simulink model "ex_longitudinal_force_balance"  (R2026a)
settings: Solver=VariableStepAuto
libraries: aerolibconvert2 x1
settings Model: Creator=doyeop  LastModifiedBy=doyeop

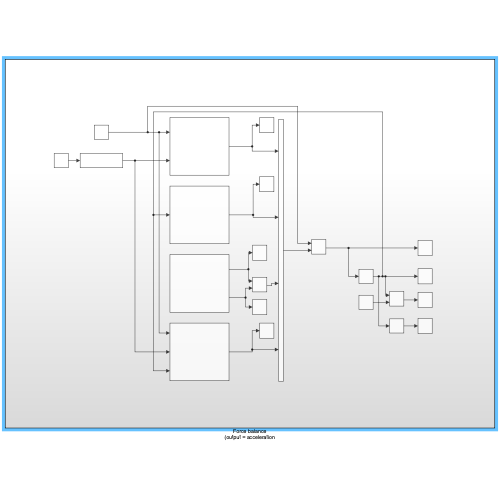
[thumbnail: Simulink's stored preview of the top-level diagram]
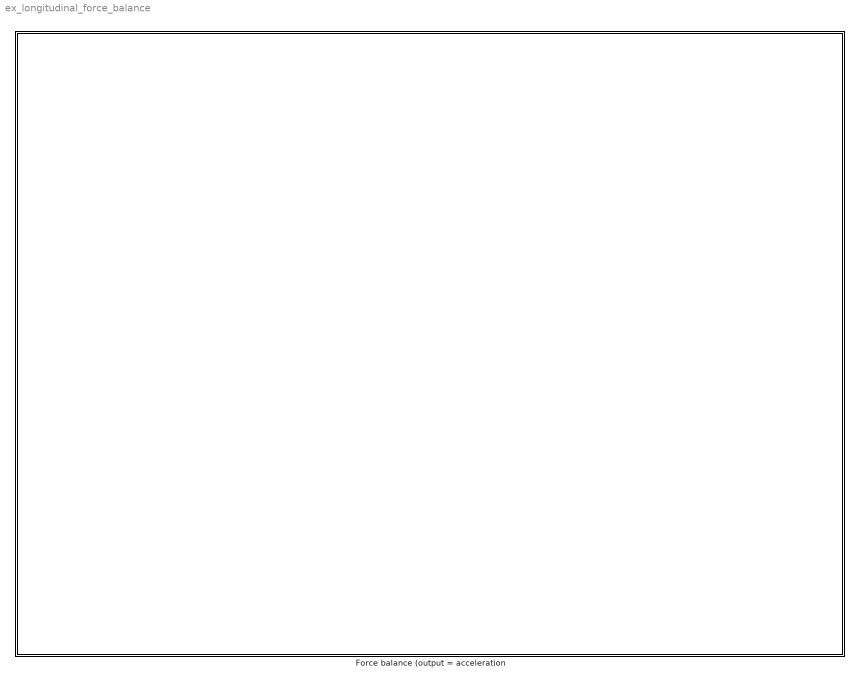
== system ex_longitudinal_force_balance ==
  Force balance (output = acceleration : Subsystem

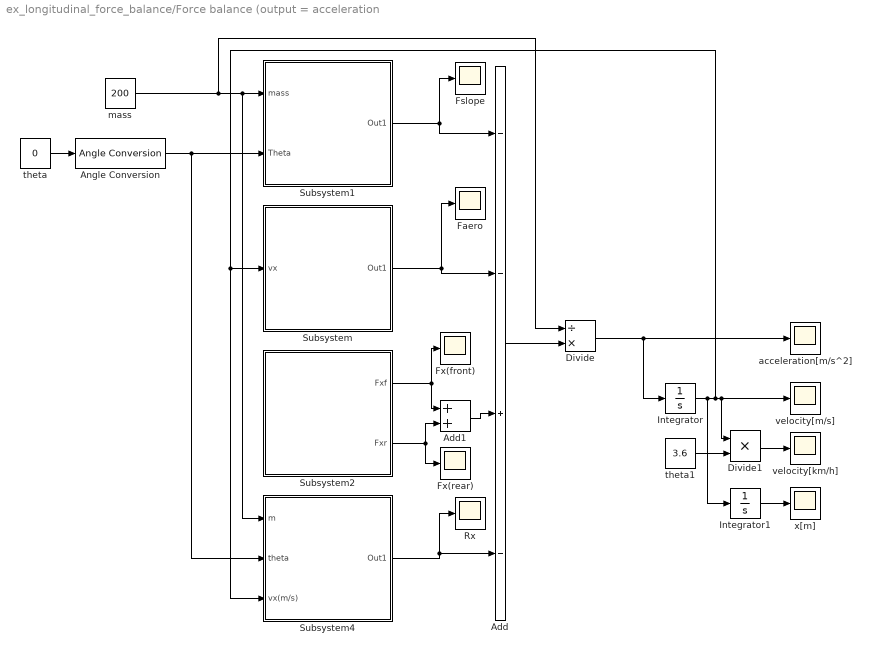
== system ex_longitudinal_force_balance/Force balance (output = acceleration ==
  Add : Sum  Inputs=--+-
  Add1 : Sum
  Angle Conversion : aerolibconvert2/Angle Conversion  IU=deg  OU=rad
  Divide : Product  Inputs=/*
  Divide1 : Product  Inputs=**
  Faero : Scope
      settings: ActiveDisplayYMinimum=-4.2362945775781089  ActiveDisplayYMaximum=75.173370603946083  DataLoggingVariableName=ScopeData4
  Fslope : Scope
      settings: ActiveDisplayYMinimum=467.68768501992645  ActiveDisplayYMaximum=4126.826484026702  DataLoggingVariableName=ScopeData3
  Fx(front) : Scope
      settings: ActiveDisplayYMinimum=-0.77322383064043154  ActiveDisplayYMaximum=0.91988628090500946  DataLoggingVariableName=ScopeData5
  Fx(rear) : Scope
      settings: ActiveDisplayYMinimum=-0.77322383064043154  ActiveDisplayYMaximum=0.91988628090500946  DataLoggingVariableName=ScopeData8
  Integrator : Integrator
  Integrator1 : Integrator
  Rx : Scope
      settings: ActiveDisplayYMinimum=6.9970576644945774  ActiveDisplayYMaximum=11.5824810195488  DataLoggingVariableName=ScopeData6
  Subsystem : Subsystem
  Subsystem1 : Subsystem
  Subsystem2 : Subsystem
  Subsystem4 : Subsystem
  acceleration[m/s^2] : Scope
      settings: ActiveDisplayYMinimum=1.2483964175329509  ActiveDisplayYMaximum=2.56967311187876
  mass : Constant  Value=200  SampleTime=-1
  theta : Constant  Value=0  SampleTime=-1
  theta1 : Constant  Value=3.6  SampleTime=-1
  velocity[km/h] : Scope
      settings: ActiveDisplayYMinimum=-8.6351088252964487  ActiveDisplayYMaximum=77.71597942766806  DataLoggingVariableName=ScopeData7
  velocity[m/s] : Scope
      settings: ActiveDisplayYMinimum=-2.4969197634620945  ActiveDisplayYMaximum=22.472277871158855
  x[m] : Scope
      settings: ActiveDisplayYMinimum=-13.639921733120476  ActiveDisplayYMaximum=122.75929559808431  DataLoggingVariableName=ScopeData2
  wires:
  Divide1/1 -> velocity[km/h]/1
  Subsystem/1(Out1) -> Faero/1, Add/2
  Integrator1/1 -> x[m]/1
  Add/1 -> Divide/2
  theta/1 -> Angle Conversion/1
  Angle Conversion/1 -> Subsystem4/2(theta), Subsystem1/2(Theta)
  Divide/1 -> Integrator/1, acceleration[m/s^2]/1
  mass/1 -> Divide/1, Subsystem4/1(m), Subsystem1/1(mass)
  Subsystem2/1(Fxf) -> Add1/1, Fx(front)/1
  theta1/1 -> Divide1/2
  Integrator/1 -> Integrator1/1, Subsystem4/3(vx(m/s)), Subsystem/1(vx), Divide1/1, velocity[m/s]/1
  Subsystem1/1(Out1) -> Fslope/1, Add/1
  Subsystem4/1(Out1) -> Add/4, Rx/1
  Subsystem2/2(Fxr) -> Fx(rear)/1, Add1/2
  Add1/1 -> Add/3

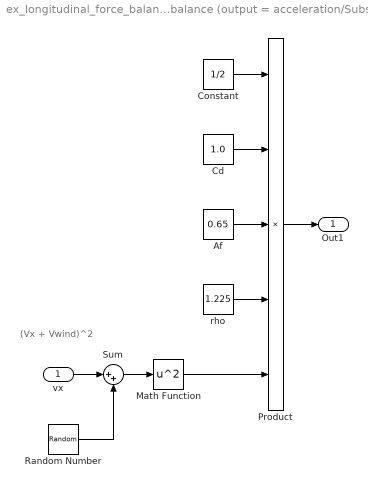
== system ex_longitudinal_force_balance/Force balance (output = acceleration/Subsystem ==
  note: (Vx + Vwind)^2
  vx : Inport
  Af : Constant  Value=0.65  SampleTime=-1
  Cd : Constant  Value=1.0  SampleTime=-1
  Constant : Constant  Value=1/2  SampleTime=-1
  Math Function : Math  Operator=square
  Product : Product  Inputs=5
  Random Number : RandomNumber  Mean=3  Variance=0.5^2  SampleTime=0.1
  Sum : Sum  Inputs=|++
  rho : Constant  Value=1.225  SampleTime=-1
  Out1 : Outport
  wires:
  Cd/1 -> Product/2
  Af/1 -> Product/3
  Constant/1 -> Product/1
  rho/1 -> Product/4
  Random Number/1 -> Sum/2
  vx/1 -> Sum/1
  Sum/1 -> Math Function/1
  Math Function/1 -> Product/5
  Product/1 -> Out1/1

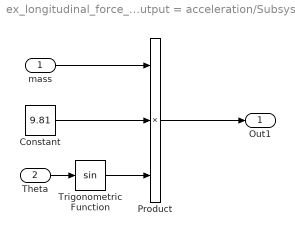
== system ex_longitudinal_force_balance/Force balance (output = acceleration/Subsystem1 ==
  mass : Inport
  Theta : Inport  Port=2
  Constant : Constant  Value=9.81  SampleTime=-1
  Product : Product  Inputs=3
  Trigonometric Function : Trigonometry
  Out1 : Outport
  wires:
  mass/1 -> Product/1
  Theta/1 -> Trigonometric Function/1
  Trigonometric Function/1 -> Product/3
  Constant/1 -> Product/2
  Product/1 -> Out1/1

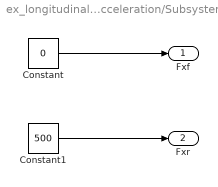
== system ex_longitudinal_force_balance/Force balance (output = acceleration/Subsystem2 ==
  Constant : Constant  Value=0  SampleTime=-1
  Constant1 : Constant  Value=500  SampleTime=-1
  Fxf : Outport
  Fxr : Outport  Port=2
  wires:
  Constant/1 -> Fxf/1
  Constant1/1 -> Fxr/1

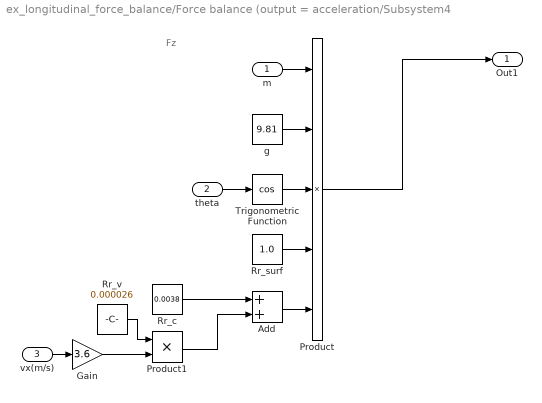
== system ex_longitudinal_force_balance/Force balance (output = acceleration/Subsystem4 ==
  note: Fz
  m : Inport
  theta : Inport  Port=2
  vx(m/s) : Inport  Port=3
  Add : Sum
  Gain : Gain  Gain=3.6
  Product : Product  Inputs=5
  Product1 : Product
  Rr_c : Constant  Value=0.0038  SampleTime=-1
  Rr_surf : Constant  Value=1.0  SampleTime=-1
  Rr_v : Constant  Value=0.000026  SampleTime=-1
  Trigonometric Function : Trigonometry  Operator=cos
  g : Constant  Value=9.81  SampleTime=-1
  Out1 : Outport
  wires:
  m/1 -> Product/1
  g/1 -> Product/2
  Trigonometric Function/1 -> Product/3
  Product/1 -> Out1/1
  theta/1 -> Trigonometric Function/1
  Rr_surf/1 -> Product/4
  Rr_v/1 -> Product1/1
  vx(m/s)/1 -> Gain/1
  Product1/1 -> Add/2
  Rr_c/1 -> Add/1
  Add/1 -> Product/5
  Gain/1 -> Product1/2
